simulink model "counter_simple"  (R2014a)
settings: Solver=FixedStepDiscrete  StartTime=0.0  StopTime=1000  FixedStep=1  RelTol=1e-3
libraries: hdlsllib x1
settings Model: Creator=you.r  LastModifiedBy=you.r

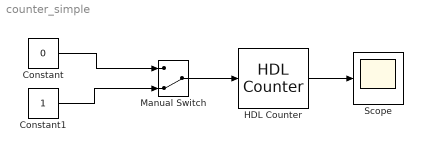
== system counter_simple ==
  Constant : Constant  Value=0  OutDataTypeStr=boolean
  Constant1 : Constant  OutDataTypeStr=boolean
  HDL Counter : hdlsllib/HDL Operations/HDL Counter  CountType=Free running  CountInit=0  CountStep=1  CountMax=100  CountFromType=Initial value  CountFrom=0  CountResetPort=off  CountLoadPort=off  CountEnbPort=on  CountDirPort=off  CountDataType=Unsigned  CountWordLen=8  CountFracLen=0  CountSampTime=1
  Manual Switch : ManualSwitch  CurrentSetting=0
  Scope : Scope
      settings: YMin=-10  YMax=10
  wires:
  Manual Switch/1 -> HDL Counter/1
  HDL Counter/1 -> Scope/1
  Constant/1 -> Manual Switch/1
  Constant1/1 -> Manual Switch/2
